simulink model "StandardModel_sl"  (Simulink 7.5)
settings: Solver=FixedStepDiscrete  StartTime=0.0  StopTime=10.0  FixedStep=0.01  RelTol=1e-3
libraries: tldummylib x8
settings Model: DS_PROJECTFILE=StandardModel.dd  TL_MAIN_DATA=struct('date',733116.453526285,'maxnumsimulations',10,'codeopt',struct('inliningthreshold',6,'target',['Generic ANSI-C'],'assembler',0,'optlevel',0,'linebreaklimit',100,'stateactcodinglimit',1,'functionsfor64bitops',1,'sections',1,'sfbitfields',1,'globalbitfields',0,'sharefunctions',0,'noinitstozero',0,'limidentlength',1,'decimals',1,'separatesearch',0,'cleancode',0,'optimizedbooltype',1,'keepsaturation',0,'extvarsharing',0,'outputstylefile','cconfig.xml','rootstylesheet','TL_CSourceCodeSS.xsl'),'frameopt',struct('exectime',1,'stacksize',1,'simconfig',['default EVM'],'targettimeout',1,'mexargs','-g','tcargs',''),'logopt',struct('plotinterval',0.1,'globalloggingmode',1),'export',struct('directory','.\export','sysfiles',1,'docfiles',0,'tools',0),'codecoveragelevel',0,'asapscript','asap2_all_in_one','docscript','tldoc_default','rtos',struct('enablemultirate',0,'currentrtos',['generic RTOS'],'autopriority',0,'autoinitalarm',1,'alarminitwithrestart',1,'alarmactivationkind',1,'alarmstartoffset',0))  Creator=alex  LastModifiedBy=alex
settings DataIOCC: SaveFormat=StructureWithTime
settings OptimizationCC: InitFltsAndDblsToZero=on
settings DebuggingCC: SaveWithParameterizedLinksMsg=none  SignalResolutionControl=TryResolveAllWithWarning  MultiTaskDSMMsg=warning  MultiTaskCondExecSysMsg=none  StrictBusMsg=None
settings RTWCC: IncludeERTFirstTime=on
settings GRTTargetCC: TargetFcnLib=ansi_tfl_tmw.mat

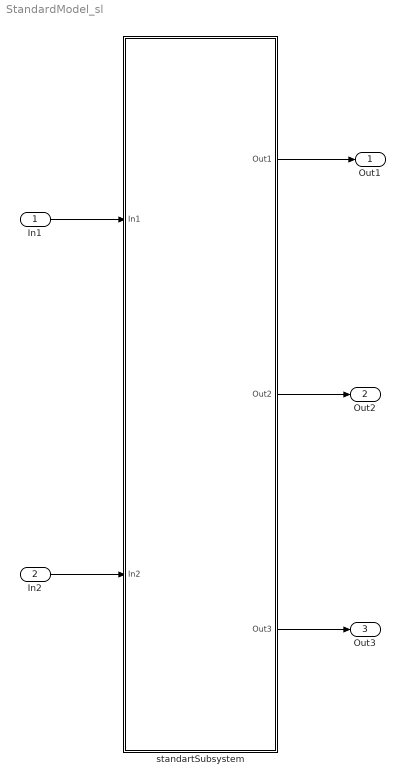
== system StandardModel_sl ==
  In1 : Inport  OutDataType=sfix(16)  OutScaling=2^0
  In2 : Inport  Port=2  OutDataType=sfix(16)  OutScaling=2^0
  standartSubsystem : Subsystem  Description=a
  Out1 : Outport  OutDataType=sfix(16)  OutScaling=2^0
  Out2 : Outport  Port=2  OutDataType=sfix(16)  OutScaling=2^0
  Out3 : Outport  Port=3  OutDataType=sfix(16)  OutScaling=2^0
  wires:
  In1/1 -> standartSubsystem/1(In1)
  In2/1 -> standartSubsystem/2(In2)
  standartSubsystem/1(Out1) -> Out1/1
  standartSubsystem/2(Out2) -> Out2/1
  standartSubsystem/3(Out3) -> Out3/1

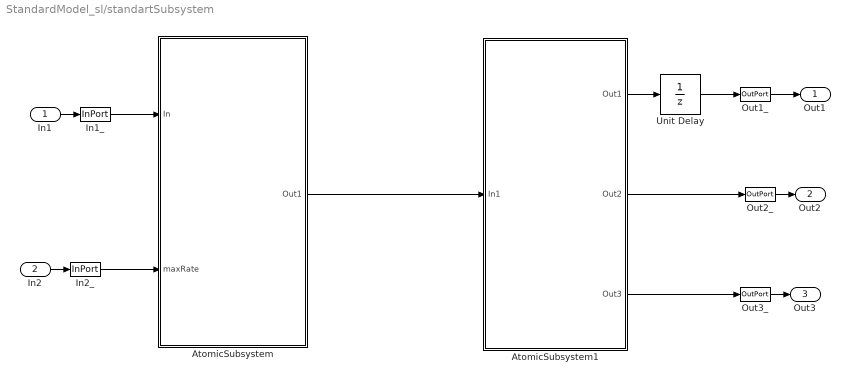
== system StandardModel_sl/standartSubsystem ==
  In1 : Inport  PortDimensions=1  OutDataType=sfix(16)  OutScaling=2^0
  In2 : Inport  Port=2  PortDimensions=1  OutDataType=sfix(16)  OutScaling=2^0
  AtomicSubsystem : Subsystem  TreatAsAtomicUnit=on
  AtomicSubsystem1 : Subsystem  TreatAsAtomicUnit=on
  In1_ : tldummylib/InPort  Tag=struct('logdata',struct('maxnumvals',inf,'plotchannels',[],'loggingmode',3,'channels',1),'output',struct('variable','','description','','name','$S_$B','width',1,'address','','max',NaN,'min',NaN,'class','default','type','Int16','scaling','','lsb',1,'offset',0,'arb',0,'freeze',1,'unit','','autoscalingmode',1,'lowerheadroom',1,'upperheadroom',1,'headroomunit','bit','keepdatatype',1,'castoutput',0,'show',0),'message',struct('name','','component','','accessor',''),'virtual',1,'scalingvalid',0,'date',733114.678131354)  SystemSampleTime=-1
  In2_ : tldummylib/InPort  Tag=struct('logdata',struct('maxnumvals',inf,'plotchannels',[],'loggingmode',3,'channels',1),'output',struct('variable','','description','','name','$S_$B','width',1,'address','','max',300,'min',-800,'class','default','type','Int16','scaling','','lsb',2^-2,'offset',-4,'arb',0,'freeze',1,'unit','','autoscalingmode',1,'lowerheadroom',1,'upperheadroom',1,'headroomunit','bit','keepdatatype',1,'castoutput',0,'show',0),'message',struct('name','','component','','accessor',''),'virtual',1,'scalingvalid',0,'date',733116.429755926)  SystemSampleTime=-1
  Out1_ : tldummylib/OutPort  Tag=struct('comment',struct('text','','placement',1),'logdata',struct('maxnumvals',inf,'plotchannels',[],'loggingmode',3,'channels',1),'output',struct('variable','','description','','name','$S_$B','width',1,'address','','max',NaN,'min',NaN,'class','default','type','Int16','scaling','','lsb',2^-1,'offset',-3,'arb',0,'freeze',1,'unit','','autoscalingmode',1,'lowerheadroom',1,'upperheadroom',1,'headroomunit','bit','keepdatatype',1,'checkmin',1,'checkmax',1,'castoutput',0,'show',0),'message',struct('name','','component',''),'virtual',0,'scalingvalid',0,'date',733116.428905822)  SystemSampleTime=-1
  Out2_ : tldummylib/OutPort  Tag=struct('comment',struct('text','','placement',1),'logdata',struct('maxnumvals',inf,'plotchannels',[],'loggingmode',3,'channels',1),'output',struct('variable','','description','','name','$S_$B','width',1,'address','','max',NaN,'min',NaN,'class','default','type','Int16','scaling','','lsb',1,'offset',0,'arb',0,'freeze',1,'unit','','autoscalingmode',1,'lowerheadroom',1,'upperheadroom',1,'headroomunit','bit','keepdatatype',1,'checkmin',0,'checkmax',0,'castoutput',0,'show',0),'message',struct('name','','component',''),'virtual',1,'scalingvalid',0,'date',733114.678132257)  SystemSampleTime=-1
  Out3_ : tldummylib/OutPort  Tag=struct('comment',struct('text','','placement',1),'logdata',struct('maxnumvals',inf,'plotchannels',[],'loggingmode',3,'channels',1),'output',struct('variable','','description','','name','$S_$B','width',1,'address','','max',NaN,'min',NaN,'class','default','type','Int32','scaling','','lsb',1,'offset',0,'arb',0,'freeze',1,'unit','','autoscalingmode',1,'lowerheadroom',1,'upperheadroom',1,'headroomunit','bit','keepdatatype',1,'checkmin',0,'checkmax',0,'castoutput',0,'show',0),'message',struct('name','','component',''),'virtual',1,'scalingvalid',0,'date',733114.678132801)  SystemSampleTime=-1
  Unit Delay : UnitDelay  Tag=struct('comment',struct('text','','placement',1),'logdata',struct('maxnumvals',inf,'plotchannels',[],'loggingmode',3,'channels',1),'output',struct('variable','','description','','name','$S_$B','width',1,'address','','max',NaN,'min',NaN,'class','default','type','Int16','scaling','','lsb',1,'offset',0,'arb',0,'freeze',1,'unit','','autoscalingmode',1,'lowerheadroom',1,'upperheadroom',1,'headroomunit','bit','keepdatatype',1,'checkmin',0,'checkmax',0,'castoutput',0,'show',0),'state',struct('variable','','description','','name','X_$S_$B','width',1,'address','','max',NaN,'min',NaN,'class','default','type','Int16','scaling','','lsb',1,'offset',0,'arb',0,'freeze',1,'unit','','initial','-2'),'dt','-1','scalingvalid',0,'date',733116.440309815)  X0=-2  SampleTime=-1
  Out1 : Outport  OutDataType=sfix(16)  OutScaling=2^0
  Out2 : Outport  Port=2  OutDataType=sfix(16)  OutScaling=2^0
  Out3 : Outport  Port=3  OutDataType=sfix(16)  OutScaling=2^0
  wires:
  Unit Delay/1 -> Out1_/1
  AtomicSubsystem1/1(Out1) -> Unit Delay/1
  AtomicSubsystem/1(Out1) -> AtomicSubsystem1/1(In1)
  In1/1 -> In1_/1
  In1_/1 -> AtomicSubsystem/1(In)
  In2/1 -> In2_/1
  In2_/1 -> AtomicSubsystem/2(maxRate)
  Out1_/1 -> Out1/1
  Out2_/1 -> Out2/1
  AtomicSubsystem1/2(Out2) -> Out2_/1
  Out3_/1 -> Out3/1
  AtomicSubsystem1/3(Out3) -> Out3_/1

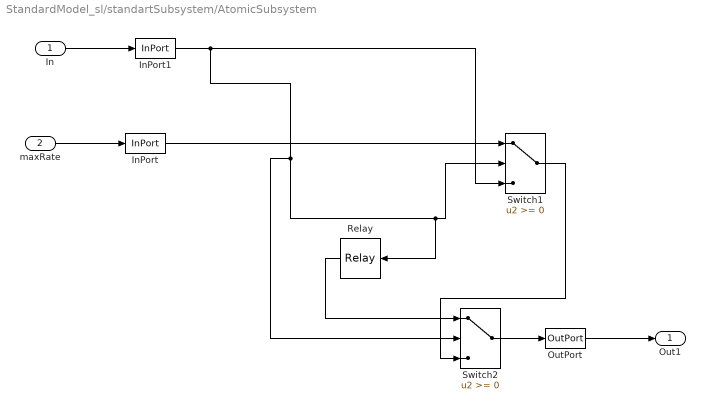
== system StandardModel_sl/standartSubsystem/AtomicSubsystem ==
  In : Inport  OutDataType=sfix(16)  OutScaling=2^0
  maxRate : Inport  Port=2  OutDataType=sfix(16)  OutScaling=2^0
  InPort : tldummylib/InPort  Tag=struct('logdata',struct('maxnumvals',inf,'plotchannels',[],'loggingmode',3,'channels',1),'output',struct('variable','','description','','name','$S_$B','width',1,'address','','max',NaN,'min',NaN,'class','FCN_REF_ARG','type','Int16','scaling','','lsb',1,'offset',0,'arb',0,'freeze',1,'unit','','autoscalingmode',1,'lowerheadroom',1,'upperheadroom',1,'headroomunit','bit','keepdatatype',1,'castoutput',0,'show',0),'message',struct('name','','component','','accessor',''),'virtual',1,'scalingvalid',0,'date',733116.436957025)  SystemSampleTime=-1
  InPort1 : tldummylib/InPort  Tag=struct('logdata',struct('maxnumvals',inf,'plotchannels',[],'loggingmode',3,'channels',1),'output',struct('variable','','description','','name','$S_$B','width',1,'address','','max',NaN,'min',NaN,'class','FCN_ARG','type','Int16','scaling','','lsb',1,'offset',0,'arb',0,'freeze',1,'unit','','autoscalingmode',1,'lowerheadroom',1,'upperheadroom',1,'headroomunit','bit','keepdatatype',1,'castoutput',0,'show',0),'message',struct('name','','component','','accessor',''),'virtual',1,'scalingvalid',0,'date',733116.437838021)  SystemSampleTime=-1
  OutPort : tldummylib/OutPort  Tag=struct('comment',struct('text','','placement',1),'logdata',struct('maxnumvals',inf,'plotchannels',[],'loggingmode',3,'channels',1),'output',struct('variable','','description','','name','$S_$B','width',1,'address','','max',NaN,'min',NaN,'class','FCN_RETURN','type','Int16','scaling','','lsb',1,'offset',0,'arb',0,'freeze',1,'unit','','autoscalingmode',1,'lowerheadroom',1,'upperheadroom',1,'headroomunit','bit','keepdatatype',1,'checkmin',0,'checkmax',0,'castoutput',0,'show',0),'message',struct('name','','component',''),'virtual',1,'scalingvalid',0,'date',733116.437082986)  SystemSampleTime=-1
  Relay : Relay  Tag=struct('comment',struct('text','','placement',1),'logdata',struct('maxnumvals',inf,'plotchannels',[],'loggingmode',3,'channels',1),'output',struct('variable','','description','','name','$S_$B','width',1,'address','','max',NaN,'min',NaN,'class','default','type','Int16','scaling','','lsb',1,'offset',0,'arb',0,'freeze',1,'unit','','autoscalingmode',1,'lowerheadroom',1,'upperheadroom',1,'headroomunit','bit','keepdatatype',1,'castoutput',0,'show',0),'onoutput',struct('variable','','description','','name','$S_$B_onoutput','width',1,'address','','max',NaN,'min',NaN,'class','CAL','type','Int16','scaling','','lsb',1,'offset',0,'arb',0,'freeze',1,'unit','','keepdatatype',1,'value','1'),'offoutput',struct('variable','','description','','name','$S_$B_offoutput','width',1,'address','','max',NaN,'min',NaN,'class','CAL','type','Int16','scaling','','lsb',1,'offset',0,'arb',0,'freeze',1,'unit','','keepdatatype',1,'value','0'),'onswitch',struct('variable','','description','','name','$S_$B_onswitch','width',1,'address','','max',NaN,'min',NaN,'class','CAL','type','Int16','scaling','','lsb',1,'offset',0,'arb',0,'freeze',1,'unit','','keepdatatype',1,'value','1','scalar',0),'offswitch',struct('variable','','description','','name','$S_$B_offswitch','width',1,'address','','max',NaN,'min',NaN,'class','CAL','type','Int16','scaling','','lsb',1,'offset',0,'arb',0,'freeze',1,'unit','','keepdatatype',1,'value','-1','scalar',0),'scalingvalid',0,'date',733110.704651296)  OnSwitchValue=1  OffSwitchValue=-1  OutDataType=sfix(16)  OutScaling=2^0
  Switch1 : Switch  Tag=struct('comment',struct('text','','placement',1),'logdata',struct('maxnumvals',inf,'plotchannels',[],'loggingmode',3,'channels',1),'output',struct('variable','','description','','name','$S_$B','width',1,'address','','max',NaN,'min',NaN,'class','default','type','Int16','scaling','','lsb',1,'offset',0,'arb',0,'freeze',1,'unit','','autoscalingmode',1,'lowerheadroom',1,'upperheadroom',1,'headroomunit','bit','keepdatatype',1,'checkmin',0,'checkmax',0,'castoutput',0,'show',0),'threshold',struct('variable','','description','','name','$S_$B_threshold','width',1,'address','','max',NaN,'min',NaN,'class','CAL','type','Int16','scaling','','lsb',1,'offset',0,'arb',0,'freeze',1,'unit','','keepdatatype',1,'value','0','scalar',0,'criteria',1),'scalingvalid',0,'date',733114.678123935)  InputSameDT=on
  Switch2 : Switch  Tag=struct('comment',struct('text','','placement',1),'logdata',struct('maxnumvals',inf,'plotchannels',[],'loggingmode',3,'channels',1),'output',struct('variable','','description','','name','$S_$B','width',1,'address','','max',NaN,'min',NaN,'class','default','type','Int16','scaling','','lsb',1,'offset',0,'arb',0,'freeze',1,'unit','','autoscalingmode',1,'lowerheadroom',1,'upperheadroom',1,'headroomunit','bit','keepdatatype',1,'checkmin',0,'checkmax',0,'castoutput',0,'show',0),'threshold',struct('variable','','description','','name','$S_$B_threshold','width',1,'address','','max',NaN,'min',NaN,'class','CAL','type','Int16','scaling','','lsb',1,'offset',0,'arb',0,'freeze',1,'unit','','keepdatatype',1,'value','0','scalar',0,'criteria',1),'scalingvalid',0,'date',733114.678124653)  InputSameDT=on
  Out1 : Outport  OutDataType=sfix(16)  OutScaling=2^0
  wires:
  InPort1/1 -> Switch2/2, Relay/1, Switch1/2, Switch1/3
  InPort/1 -> Switch1/1
  OutPort/1 -> Out1/1
  Switch2/1 -> OutPort/1
  Switch1/1 -> Switch2/3
  Relay/1 -> Switch2/1
  In/1 -> InPort1/1
  maxRate/1 -> InPort/1

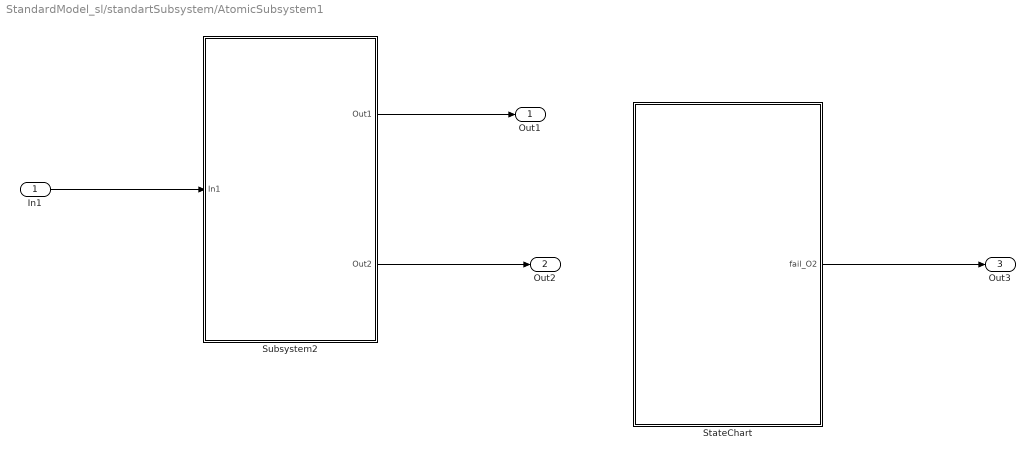
== system StandardModel_sl/standartSubsystem/AtomicSubsystem1 ==
  In1 : Inport  OutDataType=sfix(16)  OutScaling=2^0
  StateChart : Stateflow chart  Description=Stateflow diagram to determine control system operating mode  TreatAsAtomicUnit=on
  Subsystem2 : Subsystem  TreatAsAtomicUnit=on
  Out1 : Outport  OutDataType=sfix(16)  OutScaling=2^0
  Out2 : Outport  Port=2  OutDataType=sfix(16)  OutScaling=2^0
  Out3 : Outport  Port=3  OutDataType=sfix(16)  OutScaling=2^0
  wires:
  StateChart/1(fail_O2) -> Out3/1
  Subsystem2/1(Out1) -> Out1/1
  In1/1 -> Subsystem2/1(In1)
  Subsystem2/2(Out2) -> Out2/1

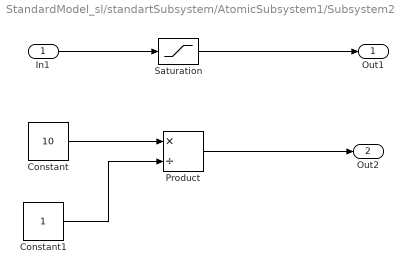
== system StandardModel_sl/standartSubsystem/AtomicSubsystem1/Subsystem2 ==
  In1 : Inport  OutDataType=sfix(16)  OutScaling=2^0
  Constant : Constant  Tag=struct('comment',struct('text','','placement',1),'output',struct('variable','','description','','name','$S_$B','width',1,'address','','max',NaN,'min',NaN,'class','GLOBAL','type','Int16','scaling','','lsb',1,'offset',0,'arb',0,'freeze',1,'unit','','keepdatatype',1,'value','10','tolerance',1,'show',0),'dt','inf','scalingvalid',0,'date',733116.443451736)  Value=10  OutDataType=sfix(16)  OutScaling=2^0
  Constant1 : Constant  Tag=struct('comment',struct('text','','placement',1),'output',struct('variable','','description','','name','$S_$B','width',1,'address','','max',NaN,'min',NaN,'class','CAL','type','Int16','scaling','','lsb',1,'offset',0,'arb',0,'freeze',1,'unit','','keepdatatype',1,'value','1','tolerance',1,'show',0),'dt','inf','scalingvalid',0,'date',733114.678125567)  OutDataType=sfix(16)  OutScaling=2^0
  Product : Product  Tag=struct('comment',struct('text','','placement',1),'logdata',struct('maxnumvals',inf,'plotchannels',[],'loggingmode',3,'channels',1),'output',struct('variable','','description','','name','$S_$B','width',1,'address','','max',NaN,'min',NaN,'class','default','type','Int16','scaling','','lsb',1,'offset',0,'arb',0,'freeze',1,'unit','','autoscalingmode',1,'lowerheadroom',1,'upperheadroom',1,'headroomunit','bit','keepdatatype',1,'checkmin',0,'checkmax',0,'castoutput',0,'show',0),'inputs','*/','exceptionhandling',1,'scalingvalid',0,'date',733116.444770463)  Inputs=*/  OutDataType=sfix(16)  OutScaling=2^0  SaturateOnIntegerOverflow=on  RndMeth=Zero  InputSameDT=on  OutDataTypeStr=Inherit: Same as first input
  Saturation : Saturate  Tag=struct('comment',struct('text','','placement',1),'logdata',struct('maxnumvals',inf,'plotchannels',[],'loggingmode',3,'channels',1),'output',struct('variable','','description','','name','$S_$B','width',1,'address','','max',255,'min',0,'class','default','type','uint16','scaling','','lsb',1,'offset',0,'arb',0,'freeze',1,'unit','','autoscalingmode',1,'lowerheadroom',1,'upperheadroom',1,'headroomunit','bit','keepdatatype',1,'castoutput',0,'show',0),'lowerlimit',struct('variable','','description','','name','$S_$B_lower','width',1,'address','','max',NaN,'min',NaN,'class','CAL','type','Int16','scaling','','lsb',1,'offset',0,'arb',0,'freeze',1,'unit','','keepdatatype',1,'value','0','scalar',0),'upperlimit',struct('variable','','description','','name','$S_$B_upper','width',1,'address','','max',NaN,'min',NaN,'class','CAL','type','Int16','scaling','','lsb',1,'offset',0,'arb',0,'freeze',1,'unit','','keepdatatype',1,'value','2','scalar',0),'scalingvalid',0,'date',733114.678127731)  UpperLimit=2  LowerLimit=0
  Out1 : Outport  OutDataType=sfix(16)  OutScaling=2^0
  Out2 : Outport  Port=2  OutDataType=sfix(16)  OutScaling=2^0
  wires:
  Product/1 -> Out2/1
  Constant/1 -> Product/1
  Constant1/1 -> Product/2
  Saturation/1 -> Out1/1
  In1/1 -> Saturation/1

== stateflow chart standartSubsystem/AtomicSubsystem1/StateChart ==
  settings: updateMethod=DISCRETE  sampleTime=0.01  description=$TL$ functionname=$O; $TL$
  state OxygenSensMode [parallel]
    settings: executionOrder=1
    settings: description=|
        | This state determines the validity of the exhaust gas oxygen sensor (EGO) data.
        | $TL$ name=$C_X_$O$R; $TL$
    state O2_Normal
      entry: fail_O2 = 0;
      settings: description=|
          | Normal EGO sensor operation gives a reliable indication of excess oxygen in the exhaust gas, from which air/fuel mixture can be inferred.
          | $TL$ name=$C_X_$O$R; $TL$
    state O2_Fail
      entry: fail_O2 = 1;
      settings: description=|
          | The EGO sensor has failed.
          | $TL$ name=$C_X_$O$R; $TL$
    state O2_Warmup
      entry: fail_O2 = 1;
      settings: description=|
          | The EGO sensor must come up to temperature before its data is reliable.
          | $TL$ name=$C_X_$O$R; $TL$
    O2_Warmup -> O2_Normal : [Calvariable== 5]
      settings: description=It is assumed that the time o2_t_thresh is sufficient for the sensor to warm up to operational temperature.
    (default) -> O2_Warmup
    O2_Normal -> O2_Fail : [Calvariable == 7]
      settings: description=The failure condition is indicated by excessive output voltage.
  data: Calvariable parameter int32 [0..1] =1; fail_O2 output int32 [0..1]
  data Calvariable settings: description=|
      | minimum manifold pressure expected at zero speed
      | $TL$ name=$C_V_$O$R; type=UInt16; lsb=2^-15; class=CAL; $TL$
  data fail_O2 settings: description=|
      | failure of oxygene sensor
      | $TL$ name=$O; type=Bool; class=MERGEABLE_DISP; $TL$
